simulink model "Simple_Joystick_HIL"  (R2025b)
settings: Solver=FixedStepDiscrete  StartTime=0.0  StopTime=tspan  FixedStep=dt_sim  RelTol=1e-3
undefined symbols (not defined in the file): dt_control, dt_data, pwm_zero_set
libraries: ros2lib x5
settings Model: Creator=vulcangrip  LastModifiedBy=vulcangrip
settings OptimizationCC: DefaultParameterBehavior=Inlined  EnhancedBackFolding=on  PassReuseOutputArgsAs=Individual arguments  ZeroExternalMemoryAtStartup=off  ZeroInternalMemoryAtStartup=off  MaxStackSize=64  OptimizeBlockOrder=speed  DifferentSizesBufferReuse=on  OptimizationCustomize=off  EfficientTunableParamExpr=on
settings DebuggingCC: ParameterTunabilityLossMsg=error
settings HardwareCC: ProdBitPerLong=64.0  ProdHWDeviceType=Intel->x86-64 (Linux 64)
settings SFSimCC: MATLABDynamicMemAlloc=off  SimTargetLang=C++  SimDLTargetLibrary=mkl-dnn
settings RTWCC: SystemTargetFile=ert.tlc  HardwareBoard=Robot Operating System 2 (ROS 2)  TLCOptions="-aInlineSetEventsForThisBaseRateFcn=TLC_FALSE -aSuppressMultiTaskScheduler=TLC_FALSE  -aRateBasedStepFcn=0"  GenCodeOnly=on  TemplateMakefile=ert_default_tmf  Toolchain=Colcon Tools  TargetLang=C++  CheckMdlBeforeBuild=Warning  Description=Embedded Coder
settings CodeAppCC: ForceParamTrailComments=on  IgnoreCustomStorageClasses=off  OperatorAnnotations=on  SimulinkDataObjDesc=on  SFDataObjDesc=on  InsertBlockDesc=on
settings ERTTargetCC: ExtModeTransport=2.0  ExtModeStaticAlloc=on  ExtModeAutomaticAllocSize=off  ExtModeMexFile=ext_xcp  ExtModeIntrfLevel=Level2 - Open  RootIOFormat=Structure reference  TargetLangStandard=C++11 (ISO)  CodeInterfacePackaging=C++ class  SubcomponentCodeInterfacePackaging=C++ class

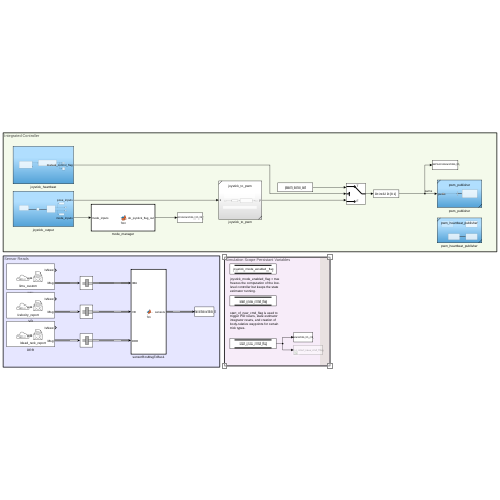
[thumbnail: Simulink's stored preview of the top-level diagram]
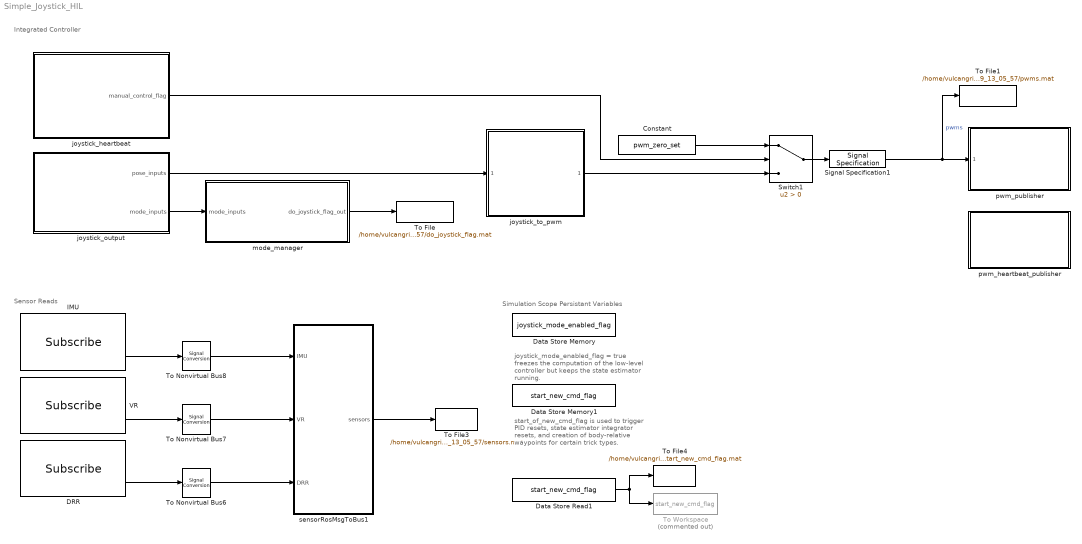
== system Simple_Joystick_HIL ==
  note: joystick_mode_enabled_flag = true freezes the computation of the low-level controller but keeps the state estimator running.
  note: Simulation Scope Persistant Variables
  note: Integrated Controller
  note: start_of_new_cmd_flag is used to trigger PID resets, state estimator integrator resets, and creation of body-relative waypoints for certain trick types.
  note: Sensor Reads
  Constant : Constant  Value=pwm_zero_set  OutDataTypeStr=int32
  DRR : ros2lib/Subscribe  topicSource=Select from ROS network  topic=/dead_reck_report  messageType=custom_interfaces/DRR  sampleTime=-1  QOSHistory=Keep last  QOSDepth=10  QOSReliability=Reliable  QOSDurability=Volatile  QOSDeadline=Inf  QOSLifespan=Inf  QOSLiveliness=Automatic  QOSLeaseDuration=Inf  QOSAvoidROSNamespaceConventions=off
  Data Store Memory : DataStoreMemory  DataStoreName=joystick_mode_enabled_flag  WriteAfterWriteMsg=warning  InitialValue=initial_joystick_mode_enabled_flag  ShowAdditionalParam=off  OutDataTypeStr=boolean
  Data Store Memory1 : DataStoreMemory  DataStoreName=start_new_cmd_flag  WriteAfterWriteMsg=warning  InitialValue=true  ShowAdditionalParam=off  OutDataTypeStr=boolean
  Data Store Read1 : DataStoreRead  DataStoreName=start_new_cmd_flag  IndexOptions=Index vector (dialog)  Indices=1  OutputSizes=1
  IMU : ros2lib/Subscribe  topicSource=Specify your own  topic=/imu_custom  messageType=custom_interfaces/Imu  sampleTime=1/100  QOSHistory=Keep last  QOSDepth=10  QOSReliability=Reliable  QOSDurability=Volatile  QOSDeadline=Inf  QOSLifespan=Inf  QOSLiveliness=Automatic  QOSLeaseDuration=Inf  QOSAvoidROSNamespaceConventions=off
  Signal Specification1 : SignalSpecification  OutDataTypeStr=int32  Dimensions=[8 1]
  Switch1 : Switch  Criteria=u2 > Threshold  SaturateOnIntegerOverflow=off  InputSameDT=off
  To File : ToFile  Filename=/home/vulcangrip/SimulinkPlant/data/2026_05_09_13_05_57/do_joystick_flag.mat  MatrixName=do_joystick_flag  SaveFormat=Timeseries  SampleTime=dt_control
  To File1 : ToFile  Filename=/home/vulcangrip/SimulinkPlant/data/2026_05_09_13_05_57/pwms.mat  MatrixName=pwms  SaveFormat=Timeseries  SampleTime=dt_control
  To File3 : ToFile  Filename=/home/vulcangrip/SimulinkPlant/data/2026_05_09_13_05_57/sensors.mat  MatrixName=sensors  SaveFormat=Timeseries
  To File4 : ToFile  Filename=/home/vulcangrip/SimulinkPlant/data/2026_05_09_13_05_57/start_new_cmd_flag.mat  MatrixName=start_new_cmd_flag  SaveFormat=Timeseries
  To Nonvirtual Bus6 : SignalConversion  ConversionOutput=Nonvirtual bus  OutDataTypeStr=Bus: SL_Bus_custom_interfaces_DRR  OverrideOpt=off
  To Nonvirtual Bus7 : SignalConversion  ConversionOutput=Nonvirtual bus  OutDataTypeStr=Bus: SL_Bus_custom_interfaces_VR  OverrideOpt=off
  To Nonvirtual Bus8 : SignalConversion  ConversionOutput=Nonvirtual bus  OutDataTypeStr=Bus: SL_Bus_custom_interfaces_Imu  OverrideOpt=off
  To Workspace : ToWorkspace  Commented=on  VariableName=start_new_cmd_flag  SaveFormat=Timeseries  SampleTime=dt_data
  VR : ros2lib/Subscribe  topicSource=Select from ROS network  topic=/velocity_report  messageType=custom_interfaces/VR  sampleTime=-1  QOSHistory=Keep last  QOSDepth=10  QOSReliability=Reliable  QOSDurability=Volatile  QOSDeadline=Inf  QOSLifespan=Inf  QOSLiveliness=Automatic  QOSLeaseDuration=Inf  QOSAvoidROSNamespaceConventions=off
  joystick_heartbeat : Subsystem
  joystick_output : Subsystem
  joystick_to_pwm : Subsystem  ReferencedSubsystem=joystick_to_pwm
  mode_manager : MATLAB Function  TreatAsAtomicUnit=on
  pwm_heartbeat_publisher : Subsystem  ReferencedSubsystem=pwm_heartbeat_publisher
  pwm_publisher : Subsystem  ReferencedSubsystem=pwm_publisher
  sensorRosMsgToBus1 : MATLAB Function  TreatAsAtomicUnit=on
  wires:
  To Nonvirtual Bus6/1 -> sensorRosMsgToBus1/3(DRR)
  joystick_to_pwm/1 -> Switch1/3
  sensorRosMsgToBus1/1(sensors) -> To File3/1
  IMU/2 -> To Nonvirtual Bus8/1
  Constant/1 -> Switch1/1
  DRR/2 -> To Nonvirtual Bus6/1
  joystick_heartbeat/1(manual_control_flag) -> Switch1/2
  Switch1/1 -> Signal Specification1/1
  VR/2 -> To Nonvirtual Bus7/1
  mode_manager/1(do_joystick_flag_out) -> To File/1
  To Nonvirtual Bus7/1 -> sensorRosMsgToBus1/2(VR)
  Data Store Read1/1 -> To File4/1, To Workspace/1
  To Nonvirtual Bus8/1 -> sensorRosMsgToBus1/1(IMU)
  joystick_output/2(mode_inputs) -> mode_manager/1(mode_inputs)
  joystick_output/1(pose_inputs) -> joystick_to_pwm/1
  Signal Specification1/1 -> pwm_publisher/1, To File1/1  "pwms"

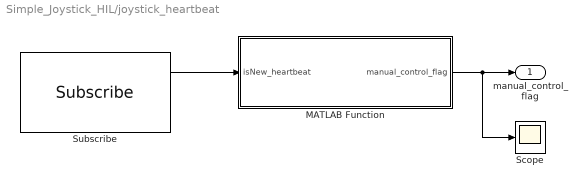
== system Simple_Joystick_HIL/joystick_heartbeat ==
  MATLAB Function : MATLAB Function  TreatAsAtomicUnit=on
  Scope : Scope
      settings: ActiveDisplayYMinimum=0.9  ActiveDisplayYMaximum=1.1
  Subscribe : ros2lib/Subscribe  topicSource=Select from ROS network  topic=/joystick_heartbeat  messageType=std_msgs/Empty  sampleTime=-1  QOSHistory=Keep last  QOSDepth=10  QOSReliability=Reliable  QOSDurability=Volatile  QOSDeadline=Inf  QOSLifespan=Inf  QOSLiveliness=Automatic  QOSLeaseDuration=Inf  QOSAvoidROSNamespaceConventions=off
  manual_control_flag : Outport
  wires:
  Subscribe/1 -> MATLAB Function/1(isNew_heartbeat)
  MATLAB Function/1(manual_control_flag) -> Scope/1, manual_control_flag/1

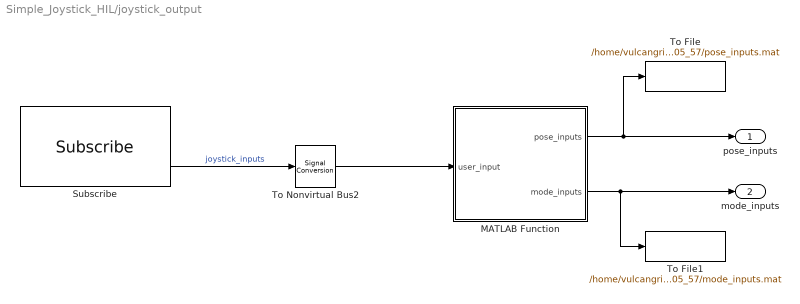
== system Simple_Joystick_HIL/joystick_output ==
  MATLAB Function : MATLAB Function  TreatAsAtomicUnit=on
  Subscribe : ros2lib/Subscribe  topicSource=Specify your own  topic=/ps5_controller  messageType=custom_interfaces/Gamepad  sampleTime=1/100  QOSHistory=Keep last  QOSDepth=10  QOSReliability=Reliable  QOSDurability=Volatile  QOSDeadline=Inf  QOSLifespan=Inf  QOSLiveliness=Automatic  QOSLeaseDuration=Inf  QOSAvoidROSNamespaceConventions=off
  To File : ToFile  Filename=/home/vulcangrip/SimulinkPlant/data/2026_05_09_13_05_57/pose_inputs.mat  MatrixName=pose_inputs  SaveFormat=Timeseries  SampleTime=dt_control
  To File1 : ToFile  Filename=/home/vulcangrip/SimulinkPlant/data/2026_05_09_13_05_57/mode_inputs.mat  MatrixName=mode_inputs  SaveFormat=Timeseries  SampleTime=dt_control
  To Nonvirtual Bus2 : SignalConversion  ConversionOutput=Nonvirtual bus  OutDataTypeStr=Bus: SL_Bus_custom_interfaces_Gamepad  OverrideOpt=off
  pose_inputs : Outport
  mode_inputs : Outport  Port=2
  wires:
  Subscribe/2 -> To Nonvirtual Bus2/1  "joystick_inputs"
  To Nonvirtual Bus2/1 -> MATLAB Function/1(user_input)
  MATLAB Function/1(pose_inputs) -> pose_inputs/1, To File/1
  MATLAB Function/2(mode_inputs) -> To File1/1, mode_inputs/1

== matlab function Simple_Joystick_HIL/joystick_heartbeat/MATLAB Function ==
  data: isNew_heartbeat input boolean; manual_control_flag output boolean; dt_control parameter
function manual_control_flag = fcn(isNew_heartbeat,dt_control)

manual_control_flag = heartbeat_interpreter(isNew_heartbeat,dt_control);

== matlab function Simple_Joystick_HIL/joystick_output/MATLAB Function ==
  data: user_input input; pose_inputs output; mode_inputs output
function [pose_inputs, mode_inputs] = fcn(user_input)

[pose_inputs, mode_inputs] = gamepad_parser(user_input);

== matlab function Simple_Joystick_HIL/mode_manager ==
  data: mode_inputs input; do_joystick_flag_out output
function do_joystick_flag_out   = fcn(mode_inputs)
    
[do_joystick_flag_out,~] = mode_manager(mode_inputs);

== matlab function Simple_Joystick_HIL/sensorRosMsgToBus1 ==
  data: IMU input; sensors output Bus: sensor_bus; VR input; DRR input size=[1,1]
function sensors = fcn(IMU, VR, DRR)

sensors = sensorRosMsgToBus(IMU, VR, DRR);
